simulink model "Flash_FCC"  (R2019b)
settings: Solver=FixedStepAuto  StartTime=0.0  StopTime=inf  RelTol=1e-3
undefined symbols (not defined in the file): Autopilot, AUX, den_lpf_d, dev, DiscIntNeverNeededParam, HIL_Data, num_lpf_d, pwm_output1
libraries: simulink_extras x4, px4lib x3, etargetslib x2, px4Sensorslib x1
settings Model: ExtModeTrigDuration=10  Creator=The MathWorks, Inc.  LastModifiedBy=guy-m
settings SolverCC: PositivePriorityOrder=on  AutoInsertRateTranBlk=on
settings OptimizationCC: EnhancedBackFolding=on  PassReuseOutputArgsAs=Individual arguments  MaxStackSize=64  OptimizeBlockOrder=speed  DifferentSizesBufferReuse=on  OptimizationCustomize=off  EfficientTunableParamExpr=on
settings DebuggingCC: InheritedTsInSrcMsg=none  ParameterTunabilityLossMsg=error
settings HardwareCC: ProdBitPerPointer=32  ProdBitPerSizeT=32  ProdBitPerPtrDiffT=32  ProdLargestAtomicInteger=Long  ProdLargestAtomicFloat=Double  ProdWordSize=32  ProdLongLongMode=on  ProdHWDeviceType=ARM Compatible->ARM Cortex
settings SFSimCC: MATLABDynamicMemAlloc=off  CustomCodeUndefinedFunction=UseInterfaceOnly
settings RTWCC: SystemTargetFile=ert.tlc  HardwareBoard=PX4 Pixhawk Series  TLCOptions="-aInlineSetEventsForThisBaseRateFcn=TLC_FALSE -aSuppressMultiTaskScheduler=TLC_FALSE  -aRateBasedStepFcn=0"  TemplateMakefile=ert_default_tmf  Toolchain=GNU Tools for PX4 Autopilots  IncludeHyperlinkInReport=on  TargetLang=C++
settings CodeAppCC: ForceParamTrailComments=on  IgnoreCustomStorageClasses=off  OperatorAnnotations=on  SimulinkDataObjDesc=on  SFDataObjDesc=on  InsertBlockDesc=on
settings ERTTargetCC: SupportContinuousTime=on  SupportVariableSizeSignals=on

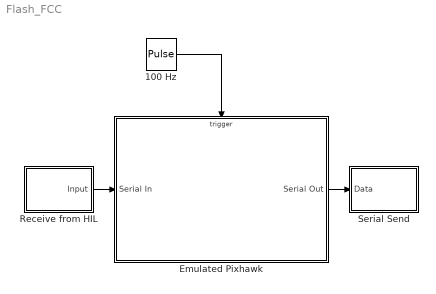
== system Flash_FCC ==
  100 Hz : DiscretePulseGenerator  PulseType=Time based  Period=0.01  PulseWidth=50
  Emulated Pixhawk : Subsystem
  Receive from HIL : Subsystem
  Serial Send : Subsystem
  wires:
  100 Hz/1 -> Emulated Pixhawk/Trigger
  Receive from HIL/1(Input) -> Emulated Pixhawk/1(Serial In)
  Emulated Pixhawk/1(Serial Out) -> Serial Send/1(Data)

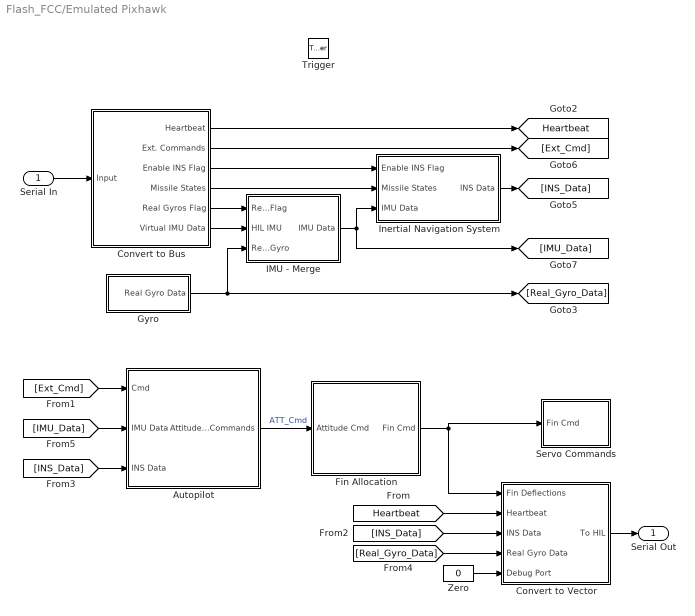
== system Flash_FCC/Emulated Pixhawk ==
  Serial In : Inport
  Trigger : TriggerPort  VariantControl=Variant  PortDimensions=1
  Autopilot : Subsystem
  Convert to Bus : Subsystem
  Convert to Vector : Subsystem
  Fin Allocation : Subsystem
  Gyro : Subsystem
  IMU - Merge : Subsystem
  Inertial Navigation System : Subsystem
  Servo Commands : Subsystem
  Zero : Constant  Value=0  OutDataTypeStr=Inherit: Inherit via back propagation
  Serial Out : Outport
  tag scope: Heartbeat=global
  wires:
  [Real_Gyro_Data] -> Convert to Vector/4(Real Gyro Data)
  Convert to Bus/2(Ext. Commands) -> [Ext_Cmd]
  Autopilot/1(Attitude_Commands) -> Fin Allocation/1(Attitude Cmd)  "ATT_Cmd"
  Convert to Bus/3(Enable INS Flag) -> Inertial Navigation System/1(Enable INS Flag)
  Inertial Navigation System/1(INS Data) -> [INS_Data]
  Zero/1 -> Convert to Vector/5(Debug Port)
  [Ext_Cmd] -> Autopilot/1(Cmd)
  [Heartbeat] -> Convert to Vector/2(Heartbeat)
  [IMU_Data] -> Autopilot/2(IMU Data)
  [INS_Data] -> Autopilot/3(INS Data)
  Gyro/1(Real Gyro Data) -> [Real_Gyro_Data], IMU - Merge/3(Real Gyro)
  IMU - Merge/1(IMU Data) -> [IMU_Data], Inertial Navigation System/3(IMU Data)
  Convert to Vector/1(To HIL) -> Serial Out/1
  Fin Allocation/1(Fin Cmd) -> Servo Commands/1(Fin Cmd), Convert to Vector/1(Fin Deflections)
  Serial In/1 -> Convert to Bus/1(Input)
  [INS_Data] -> Convert to Vector/3(INS Data)
  Convert to Bus/5(Real Gyros Flag) -> IMU - Merge/1(Real Gyro Flag)
  Convert to Bus/4(Missile States) -> Inertial Navigation System/2(Missile States)
  Convert to Bus/1(Heartbeat) -> [Heartbeat]
  Convert to Bus/6(Virtual IMU Data) -> IMU - Merge/2(HIL IMU)

== system Flash_FCC/Receive from HIL ==
  NOT : Logic  Operator=NOT  IconShape=distinctive  AllPortsSameDT=off  OutDataTypeStr=boolean
  Serial Receive : px4lib/Serial Receive  SCIModule=/dev/ttyACM0  DataType=single  DataLength=23  OutputStatus=on  SampleTime=0.001  BlockingMode=off  PartialData=off  Timeout=5
      settings: SourceProductName=Embedded Coder Support Package for PX4 Autopilots  SourceProductBaseCode=PX4AUTOPILOTS
  Triggered Subsystem : Subsystem  TreatAsAtomicUnit=on
  Input : Outport
  wires:
  Serial Receive/2 -> NOT/1
  NOT/1 -> Triggered Subsystem/Trigger
  Serial Receive/1 -> Triggered Subsystem/1(In1)
  Triggered Subsystem/1(Out1) -> Input/1

== system Flash_FCC/Serial Send ==
  Data : Inport
  Byte Pack : etargetslib/Byte Pack  datatypes={'single'}  byteAlign=1
      settings: SourceProductName=MATLAB Coder
  Header : Subsystem
  Serial Transmit : px4lib/Serial Transmit  SCIModule=/dev/ttyACM0
      settings: SourceProductName=Embedded Coder Support Package for PX4 Autopilots  SourceProductBaseCode=PX4AUTOPILOTS
  Vector Concatenate1 : Concatenate
  wires:
  Header/1(Out1) -> Vector Concatenate1/1
  Vector Concatenate1/1 -> Serial Transmit/1
  Byte Pack/1 -> Vector Concatenate1/2
  Data/1 -> Byte Pack/1

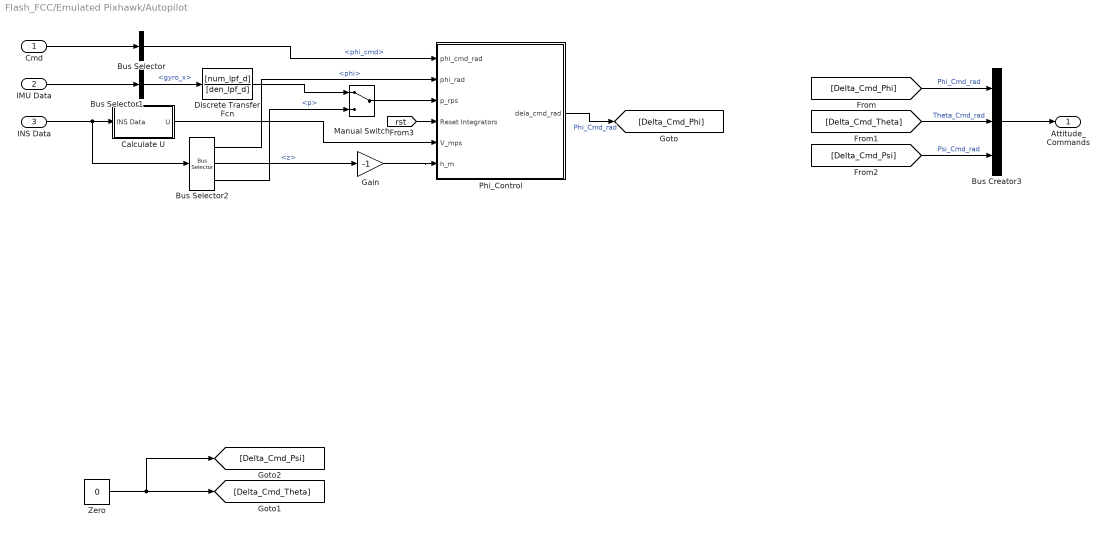
== system Flash_FCC/Emulated Pixhawk/Autopilot ==
  Cmd : Inport
  IMU Data : Inport  Port=2
  INS Data : Inport  Port=3
  Bus Creator3 : BusCreator  Inputs=3
  Bus Selector : BusSelector  OutputSignals=phi_cmd
  Bus Selector1 : BusSelector  OutputSignals=gyro_x
  Bus Selector2 : BusSelector  OutputSignals=phi,z,p
  Calculate U : Subsystem
  Discrete Transfer Fcn : DiscreteTransferFcn  Numerator=[num_lpf_d]  Denominator=[den_lpf_d]
  Gain : Gain  Gain=-1
  Manual Switch : ManualSwitch
  Phi_Control : Subsystem
  Zero : Constant  Value=0  OutDataTypeStr=Inherit: Inherit via back propagation
  Attitude_Commands : Outport  VectorParamsAs1DForOutWhenUnconnected=off
  wires:
  Bus Selector1/1 -> Discrete Transfer Fcn/1  "<gyro_x>"
  IMU Data/1 -> Bus Selector1/1
  Calculate U/1(U) -> Phi_Control/5(V_mps)
  Zero/1 -> [Delta_Cmd_Psi], [Delta_Cmd_Theta]
  [Delta_Cmd_Phi] -> Bus Creator3/1  "Phi_Cmd_rad"
  [Delta_Cmd_Theta] -> Bus Creator3/2  "Theta_Cmd_rad"
  Bus Creator3/1 -> Attitude_Commands/1
  [Delta_Cmd_Psi] -> Bus Creator3/3  "Psi_Cmd_rad"
  Bus Selector/1 -> Phi_Control/1(phi_cmd_rad)  "<phi_cmd>"
  Cmd/1 -> Bus Selector/1
  INS Data/1 -> Calculate U/1(INS Data), Bus Selector2/1
  Bus Selector2/1 -> Phi_Control/2(phi_rad)  "<phi>"
  [rst] -> Phi_Control/4(Reset Integrators)
  Bus Selector2/2 -> Gain/1  "<z>"
  Gain/1 -> Phi_Control/6(h_m)
  Phi_Control/1(dela_cmd_rad) -> [Delta_Cmd_Phi]  "Phi_Cmd_rad"
  Discrete Transfer Fcn/1 -> Manual Switch/1
  Bus Selector2/3 -> Manual Switch/2  "<p>"
  Manual Switch/1 -> Phi_Control/3(p_rps)

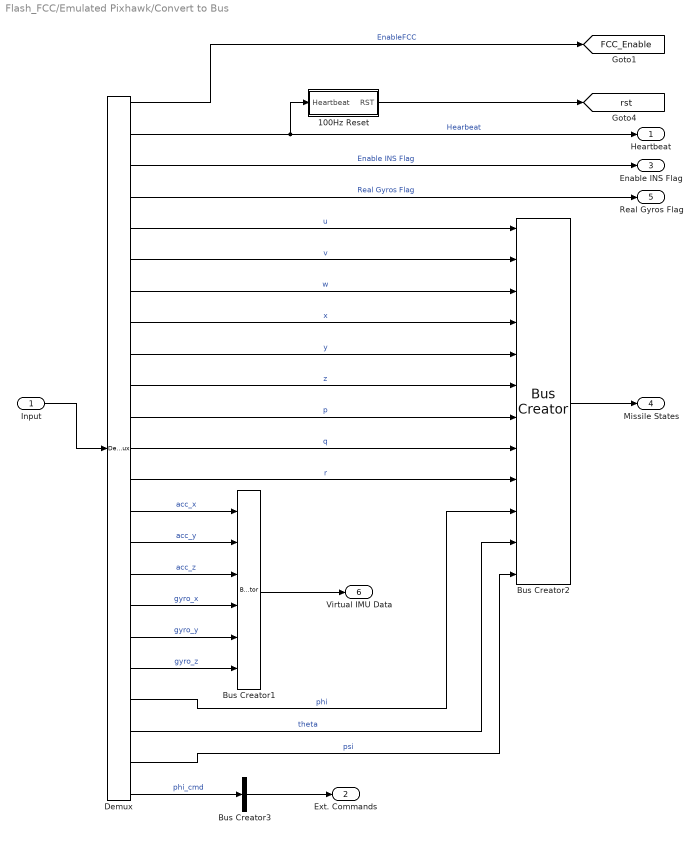
== system Flash_FCC/Emulated Pixhawk/Convert to Bus ==
  Input : Inport  OutDataTypeStr=single
  100Hz Reset : Subsystem
  Bus Creator1 : BusCreator  Inputs=6
  Bus Creator2 : BusCreator  Inputs=12
  Bus Creator3 : BusCreator  Inputs=1
  Demux : Demux  Outputs=23
  Heartbeat : Outport  InitialOutput=0
  Ext. Commands : Outport  Port=2  OutDataTypeStr=single  InitialOutput=0
  Enable INS Flag : Outport  Port=3  InitialOutput=0
  Missile States : Outport  Port=4  OutDataTypeStr=single  InitialOutput=[0 0 0 0 0 0 0 0 0 0]
  Real Gyros Flag : Outport  Port=5  InitialOutput=0
  Virtual IMU Data : Outport  Port=6  OutDataTypeStr=single  InitialOutput=[0 0 0 0 0 0 0 0 0 0]
  tag scope: FCC_Enable=global, rst=global
  wires:
  Demux/22 -> Bus Creator2/12  "psi"
  Demux/21 -> Bus Creator2/11  "theta"
  Demux/20 -> Bus Creator2/10  "phi"
  Demux/4 -> Real Gyros Flag/1  "Real Gyros Flag"
  Demux/5 -> Bus Creator2/1  "u"
  Demux/18 -> Bus Creator1/5  "gyro_y"
  Bus Creator1/1 -> Virtual IMU Data/1
  Demux/16 -> Bus Creator1/3  "acc_z"
  Demux/9 -> Bus Creator2/5  "y"
  Demux/14 -> Bus Creator1/1  "acc_x"
  Demux/17 -> Bus Creator1/4  "gyro_x"
  Demux/15 -> Bus Creator1/2  "acc_y"
  Demux/19 -> Bus Creator1/6  "gyro_z"
  Demux/12 -> Bus Creator2/8  "q"
  Demux/7 -> Bus Creator2/3  "w"
  Demux/10 -> Bus Creator2/6  "z"
  Demux/6 -> Bus Creator2/2  "v"
  Demux/11 -> Bus Creator2/7  "p"
  Demux/13 -> Bus Creator2/9  "r"
  Demux/23 -> Bus Creator3/1  "phi_cmd"
  Demux/8 -> Bus Creator2/4  "x"
  Bus Creator3/1 -> Ext. Commands/1
  Bus Creator2/1 -> Missile States/1
  Demux/1 -> [FCC_Enable]  "EnableFCC"
  Input/1 -> Demux/1
  Demux/2 -> 100Hz Reset/1(Heartbeat), Heartbeat/1  "Hearbeat"
  Demux/3 -> Enable INS Flag/1  "Enable INS Flag"
  100Hz Reset/1(RST) -> [rst]

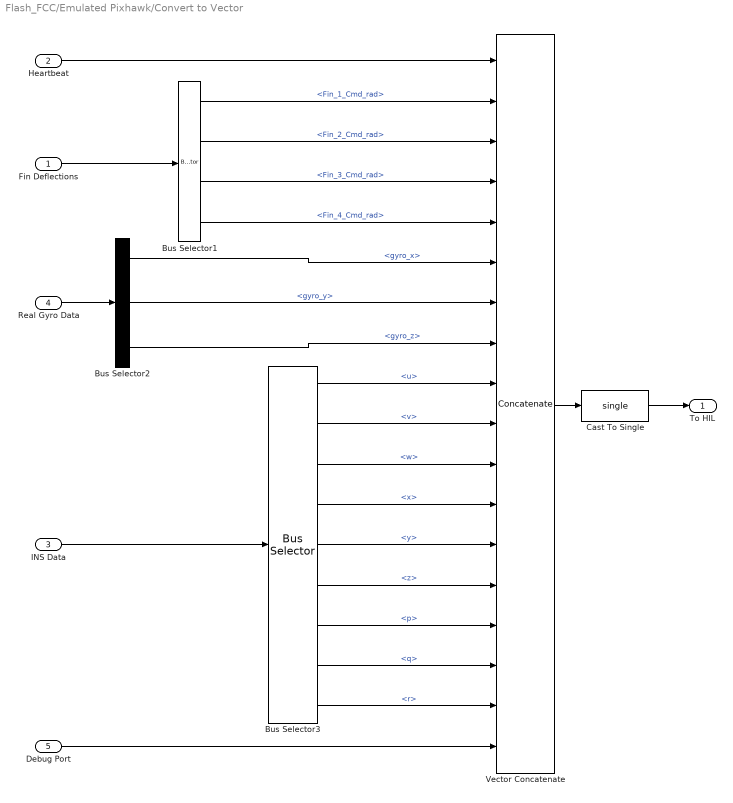
== system Flash_FCC/Emulated Pixhawk/Convert to Vector ==
  Fin Deflections : Inport
  Heartbeat : Inport  Port=2
  INS Data : Inport  Port=3
  Real Gyro Data : Inport  Port=4
  Debug Port : Inport  Port=5
  Bus Selector1 : BusSelector  OutputSignals=Fin_1_Cmd_rad,Fin_2_Cmd_rad,Fin_3_Cmd_rad,Fin_4_Cmd_rad
  Bus Selector2 : BusSelector  OutputSignals=gyro_x,gyro_y,gyro_z
  Bus Selector3 : BusSelector  OutputSignals=u,v,w,x,y,z,p,q,r
  Cast To Single : DataTypeConversion  OutDataTypeStr=single
  Vector Concatenate : Concatenate  NumInputs=18
  To HIL : Outport
  wires:
  Bus Selector1/3 -> Vector Concatenate/4  "<Fin_3_Cmd_rad>"
  Bus Selector1/4 -> Vector Concatenate/5  "<Fin_4_Cmd_rad>"
  Heartbeat/1 -> Vector Concatenate/1
  Bus Selector1/1 -> Vector Concatenate/2  "<Fin_1_Cmd_rad>"
  Bus Selector1/2 -> Vector Concatenate/3  "<Fin_2_Cmd_rad>"
  Vector Concatenate/1 -> Cast To Single/1
  Fin Deflections/1 -> Bus Selector1/1
  Cast To Single/1 -> To HIL/1
  Real Gyro Data/1 -> Bus Selector2/1
  Bus Selector3/7 -> Vector Concatenate/15  "<p>"
  Bus Selector3/5 -> Vector Concatenate/13  "<y>"
  Bus Selector3/4 -> Vector Concatenate/12  "<x>"
  Bus Selector3/9 -> Vector Concatenate/17  "<r>"
  Bus Selector3/3 -> Vector Concatenate/11  "<w>"
  Bus Selector2/3 -> Vector Concatenate/8  "<gyro_z>"
  Debug Port/1 -> Vector Concatenate/18
  Bus Selector3/1 -> Vector Concatenate/9  "<u>"
  Bus Selector2/2 -> Vector Concatenate/7  "<gyro_y>"
  Bus Selector2/1 -> Vector Concatenate/6  "<gyro_x>"
  Bus Selector3/8 -> Vector Concatenate/16  "<q>"
  INS Data/1 -> Bus Selector3/1
  Bus Selector3/6 -> Vector Concatenate/14  "<z>"
  Bus Selector3/2 -> Vector Concatenate/10  "<v>"

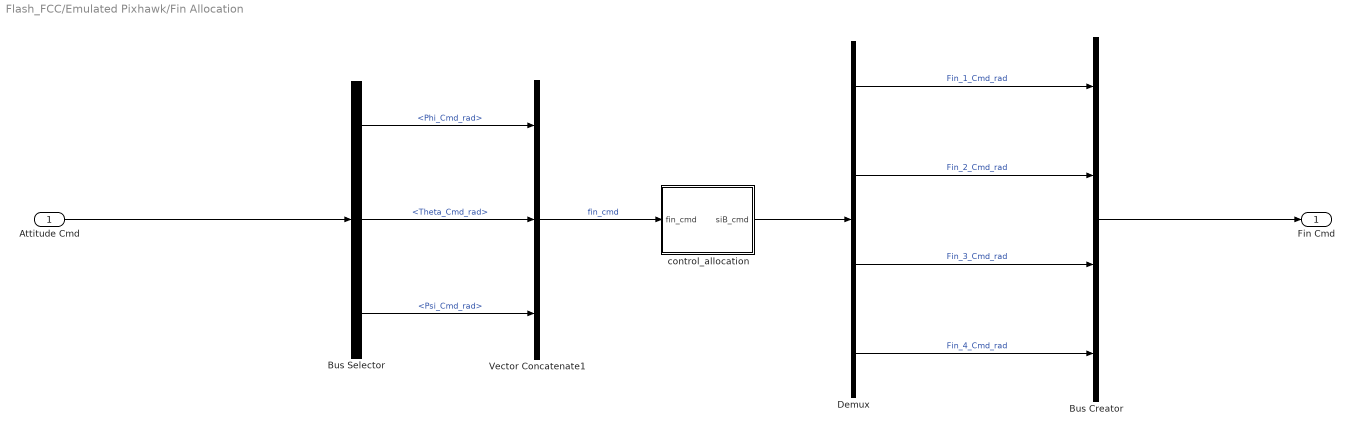
== system Flash_FCC/Emulated Pixhawk/Fin Allocation ==
  Attitude Cmd : Inport
  Bus Creator : BusCreator  Inputs=4
  Bus Selector : BusSelector  OutputSignals=Phi_Cmd_rad,Theta_Cmd_rad,Psi_Cmd_rad
  Demux : Demux
  Vector Concatenate1 : Concatenate  NumInputs=3
  control_allocation : Subsystem
  Fin Cmd : Outport  VectorParamsAs1DForOutWhenUnconnected=off
  wires:
  Demux/4 -> Bus Creator/4  "Fin_4_Cmd_rad"
  control_allocation/1(siB_cmd) -> Demux/1
  Bus Selector/3 -> Vector Concatenate1/3  "<Psi_Cmd_rad>"
  Vector Concatenate1/1 -> control_allocation/1(fin_cmd)  "fin_cmd"
  Bus Selector/1 -> Vector Concatenate1/1  "<Phi_Cmd_rad>"
  Demux/3 -> Bus Creator/3  "Fin_3_Cmd_rad"
  Bus Selector/2 -> Vector Concatenate1/2  "<Theta_Cmd_rad>"
  Demux/1 -> Bus Creator/1  "Fin_1_Cmd_rad"
  Bus Creator/1 -> Fin Cmd/1
  Attitude Cmd/1 -> Bus Selector/1
  Demux/2 -> Bus Creator/2  "Fin_2_Cmd_rad"

== system Flash_FCC/Emulated Pixhawk/Gyro ==
  Bus Creator2 : BusCreator  Inputs=3
  Gyroscope : px4Sensorslib/Gyroscope  uorbTimeStamp=off  BlockingMode=off  BlockTimeout=1e-3  sampleTime=-1
      settings: SourceProductName=Embedded Coder Support Package for PX4 Autopilots  SourceProductBaseCode=PX4AUTOPILOTS
  Terminator3 : Terminator
  Real Gyro Data : Outport
  wires:
  Gyroscope/1 -> Terminator3/1
  Bus Creator2/1 -> Real Gyro Data/1  "gyro"
  Gyroscope/4 -> Bus Creator2/3  "gyro_z"
  Gyroscope/2 -> Bus Creator2/1  "gyro_x"
  Gyroscope/3 -> Bus Creator2/2  "gyro_y"

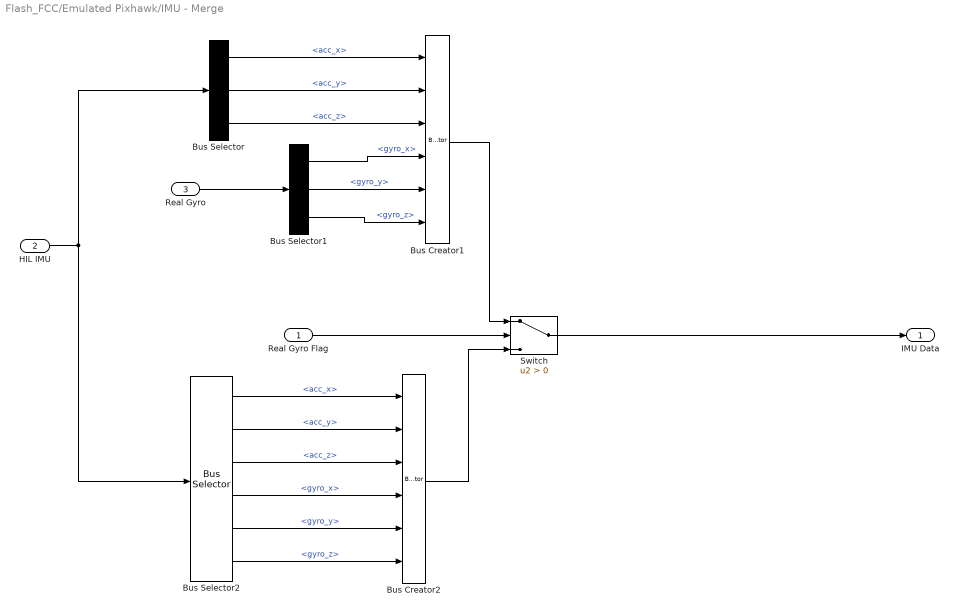
== system Flash_FCC/Emulated Pixhawk/IMU - Merge ==
  Real Gyro Flag : Inport
  HIL IMU : Inport  Port=2
  Real Gyro : Inport  Port=3
  Bus Creator1 : BusCreator  Inputs=6
  Bus Creator2 : BusCreator  Inputs=6
  Bus Selector : BusSelector  OutputSignals=acc_x,acc_y,acc_z
  Bus Selector1 : BusSelector  OutputSignals=gyro_x,gyro_y,gyro_z
  Bus Selector2 : BusSelector  OutputSignals=acc_x,acc_y,acc_z,gyro_x,gyro_y,gyro_z
  Switch : Switch  Criteria=u2 > Threshold
  IMU Data : Outport
  wires:
  Real Gyro Flag/1 -> Switch/2
  Real Gyro/1 -> Bus Selector1/1
  HIL IMU/1 -> Bus Selector2/1, Bus Selector/1
  Bus Selector/3 -> Bus Creator1/3  "<acc_z>"
  Bus Selector/1 -> Bus Creator1/1  "<acc_x>"
  Bus Selector/2 -> Bus Creator1/2  "<acc_y>"
  Bus Selector1/1 -> Bus Creator1/4  "<gyro_x>"
  Bus Selector1/3 -> Bus Creator1/6  "<gyro_z>"
  Bus Creator1/1 -> Switch/1
  Bus Selector1/2 -> Bus Creator1/5  "<gyro_y>"
  Bus Selector2/5 -> Bus Creator2/5  "<gyro_y>"
  Bus Selector2/6 -> Bus Creator2/6  "<gyro_z>"
  Bus Selector2/4 -> Bus Creator2/4  "<gyro_x>"
  Bus Selector2/2 -> Bus Creator2/2  "<acc_y>"
  Bus Selector2/1 -> Bus Creator2/1  "<acc_x>"
  Bus Selector2/3 -> Bus Creator2/3  "<acc_z>"
  Bus Creator2/1 -> Switch/3
  Switch/1 -> IMU Data/1

== system Flash_FCC/Emulated Pixhawk/Inertial Navigation System ==
  Enable INS Flag : Inport
  Missile States : Inport  Port=2
  IMU Data : Inport  Port=3
  INS (INCOMPLETE) : Subsystem
  Switch : Switch  Criteria=u2 > Threshold
  INS Data : Outport
  wires:
  Enable INS Flag/1 -> Switch/2
  IMU Data/1 -> INS (INCOMPLETE)/1(IMU Data)
  Switch/1 -> INS Data/1
  Missile States/1 -> Switch/3
  INS (INCOMPLETE)/1(INS Data) -> Switch/1

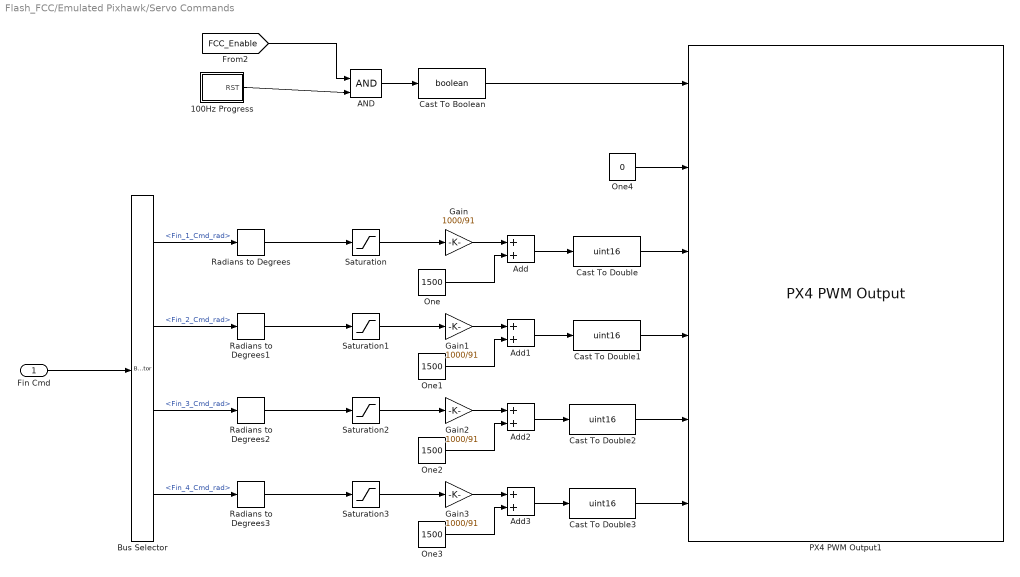
== system Flash_FCC/Emulated Pixhawk/Servo Commands ==
  Fin Cmd : Inport
  100Hz Progress : Subsystem
  AND : Logic  IconShape=distinctive  AllPortsSameDT=off  OutDataTypeStr=boolean
  Add{,1..3} (4 alike) : Sum
  Bus Selector : BusSelector  OutputSignals=Fin_1_Cmd_rad,Fin_2_Cmd_rad,Fin_3_Cmd_rad,Fin_4_Cmd_rad
  Cast To Boolean : DataTypeConversion  OutDataTypeStr=boolean
  Cast To Double{,1..3} (4 alike) : DataTypeConversion  OutDataTypeStr=uint16
  Gain{,1..3} (4 alike) : Gain  Gain=1000/91
  One{,1..3} (4 alike) : Constant  Value=1500  OutDataTypeStr=Inherit: Inherit via back propagation
  One4 : Constant  Value=0  OutDataTypeStr=boolean
  PX4 PWM Output1 : px4lib/PX4 PWM Output  pwmDevice=AUX (/dev/pwm_output1)  pwmChannel1_=on  pwmChannel2_=on  pwmChannel3_=on  pwmChannel4_=on  pwmChannel5_=off  pwmChannel6_=off  pwmChannel7_=off  pwmChannel8_=off  forceTerminateFailsafe=off  outputErrorStatus=off
      settings: SourceProductName=Embedded Coder Support Package for PX4 Autopilots  SourceProductBaseCode=PX4AUTOPILOTS
  Radians to Degrees{,1..3} (4 alike) : simulink_extras/Transformations/Radians to Degrees
  Saturation{,1..3} (4 alike) : Saturate  UpperLimit=20  LowerLimit=-20
  wires:
  Saturation2/1 -> Gain2/1
  Cast To Double3/1 -> PX4 PWM Output1/6
  One4/1 -> PX4 PWM Output1/2
  One/1 -> Add/2
  One2/1 -> Add2/2
  Add1/1 -> Cast To Double1/1
  Gain2/1 -> Add2/1
  AND/1 -> Cast To Boolean/1
  Radians to Degrees1/1 -> Saturation1/1
  Cast To Double2/1 -> PX4 PWM Output1/5
  Add2/1 -> Cast To Double2/1
  Fin Cmd/1 -> Bus Selector/1
  Cast To Double1/1 -> PX4 PWM Output1/4
  Bus Selector/2 -> Radians to Degrees1/1  "<Fin_2_Cmd_rad>"
  Gain/1 -> Add/1
  Bus Selector/4 -> Radians to Degrees3/1  "<Fin_4_Cmd_rad>"
  One3/1 -> Add3/2
  Saturation/1 -> Gain/1
  Gain1/1 -> Add1/1
  Saturation3/1 -> Gain3/1
  Gain3/1 -> Add3/1
  Radians to Degrees3/1 -> Saturation3/1
  Bus Selector/1 -> Radians to Degrees/1  "<Fin_1_Cmd_rad>"
  Bus Selector/3 -> Radians to Degrees2/1  "<Fin_3_Cmd_rad>"
  Saturation1/1 -> Gain1/1
  Cast To Double/1 -> PX4 PWM Output1/3
  Add3/1 -> Cast To Double3/1
  Radians to Degrees2/1 -> Saturation2/1
  [FCC_Enable] -> AND/1
  Radians to Degrees/1 -> Saturation/1
  100Hz Progress/1(RST) -> AND/2
  One1/1 -> Add1/2
  Add/1 -> Cast To Double/1
  Cast To Boolean/1 -> PX4 PWM Output1/1

== system Flash_FCC/Receive from HIL/Triggered Subsystem ==
  In1 : Inport
  Trigger : TriggerPort  VariantControl=Variant
  Out1 : Outport  InitialOutput=0
  wires:
  In1/1 -> Out1/1

== system Flash_FCC/Serial Send/Header ==
  note: Serial header - used to preserve order of bytes
  Byte Pack1 : etargetslib/Byte Pack  datatypes={'uint8'}  byteAlign=1
      settings: SourceProductName=MATLAB Coder
  Zero : Constant  Value=[5 5 5]  OutDataTypeStr=uint8  SampleTime=-1
  Out1 : Outport
  wires:
  Zero/1 -> Byte Pack1/1
  Byte Pack1/1 -> Out1/1

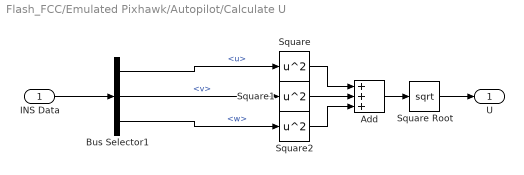
== system Flash_FCC/Emulated Pixhawk/Autopilot/Calculate U ==
  INS Data : Inport
  Add : Sum  Inputs=+++
  Bus Selector1 : BusSelector  OutputSignals=u,v,w
  Square : Math  Operator=square  SignedPower=off  SaturateOnIntegerOverflow=on
  Square Root : Sqrt  SaturateOnIntegerOverflow=on
  Square1 : Math  Operator=square  SignedPower=off  SaturateOnIntegerOverflow=on
  Square2 : Math  Operator=square  SignedPower=off  SaturateOnIntegerOverflow=on
  U : Outport
  wires:
  Square/1 -> Add/1
  Square2/1 -> Add/3
  Square Root/1 -> U/1
  Add/1 -> Square Root/1
  Square1/1 -> Add/2
  Bus Selector1/2 -> Square1/1  "<v>"
  Bus Selector1/3 -> Square2/1  "<w>"
  Bus Selector1/1 -> Square/1  "<u>"
  INS Data/1 -> Bus Selector1/1

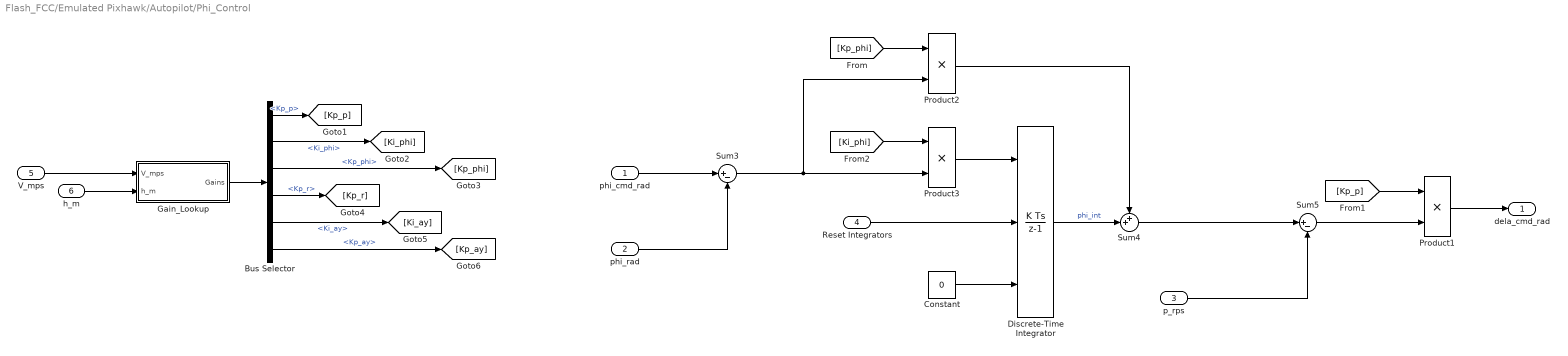
== system Flash_FCC/Emulated Pixhawk/Autopilot/Phi_Control ==
  phi_cmd_rad : Inport
  phi_rad : Inport  Port=2
  p_rps : Inport  Port=3
  Reset Integrators : Inport  Port=4
  V_mps : Inport  Port=5
  h_m : Inport  Port=6
  Bus Selector : BusSelector  OutputSignals=Kp_p,Ki_phi,Kp_phi,Kp_r,Ki_ay,Kp_ay
  Constant : Constant  Value=0  OutDataTypeStr=single
  Discrete-Time Integrator : DiscreteIntegrator  ExternalReset=level  InitialConditionSource=external  SampleTime=-1  OutDataTypeStr=single  ICPrevOutput=DiscIntNeverNeededParam  ICPrevScaledInput=DiscIntNeverNeededParam
  Gain_Lookup : Subsystem
  Product1 : Product
  Product2 : Product
  Product3 : Product
  Sum3 : Sum  Inputs=|+-
  Sum4 : Sum  Inputs=++|
  Sum5 : Sum  Inputs=|+-
  dela_cmd_rad : Outport
  wires:
  phi_cmd_rad/1 -> Sum3/1
  Reset Integrators/1 -> Discrete-Time Integrator/2
  p_rps/1 -> Sum5/2
  phi_rad/1 -> Sum3/2
  Product2/1 -> Sum4/1
  Sum3/1 -> Product3/2, Product2/2
  Constant/1 -> Discrete-Time Integrator/3
  Sum5/1 -> Product1/2
  [Ki_phi] -> Product3/1
  Product1/1 -> dela_cmd_rad/1
  [Kp_p] -> Product1/1
  [Kp_phi] -> Product2/1
  Discrete-Time Integrator/1 -> Sum4/2  "phi_int"
  Sum4/1 -> Sum5/1
  Product3/1 -> Discrete-Time Integrator/1
  h_m/1 -> Gain_Lookup/2(h_m)
  Bus Selector/6 -> [Kp_ay]  "<Kp_ay>"
  Bus Selector/5 -> [Ki_ay]  "<Ki_ay>"
  Bus Selector/2 -> [Ki_phi]  "<Ki_phi>"
  Bus Selector/1 -> [Kp_p]  "<Kp_p>"
  V_mps/1 -> Gain_Lookup/1(V_mps)
  Bus Selector/4 -> [Kp_r]  "<Kp_r>"
  Gain_Lookup/1(Gains) -> Bus Selector/1
  Bus Selector/3 -> [Kp_phi]  "<Kp_phi>"

== system Flash_FCC/Emulated Pixhawk/Convert to Bus/100Hz Reset ==
  Heartbeat : Inport
  Delay : Delay  DelayLength=1
  GreaterThan : RelationalOperator  Operator=<  OutDataTypeStr=boolean  RndMeth=Simplest
  RST : Outport
  wires:
  GreaterThan/1 -> RST/1
  Delay/1 -> GreaterThan/2
  Heartbeat/1 -> Delay/1, GreaterThan/1

== system Flash_FCC/Emulated Pixhawk/Fin Allocation/control_allocation ==
  fin_cmd : Inport
  Constant7 : Constant  Value=HIL_Data.FDM.Tr4r3  OutDataTypeStr=single
  Product : Product  Multiplication=Matrix(*)
  siB_cmd : Outport  VectorParamsAs1DForOutWhenUnconnected=off
  wires:
  Constant7/1 -> Product/1
  fin_cmd/1 -> Product/2
  Product/1 -> siB_cmd/1  "siB_cmd"

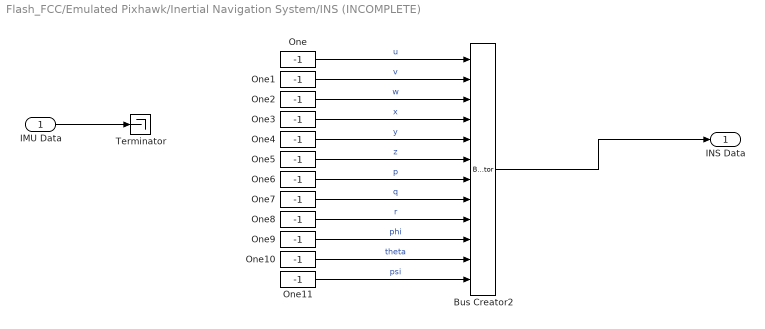
== system Flash_FCC/Emulated Pixhawk/Inertial Navigation System/INS (INCOMPLETE) ==
  IMU Data : Inport
  Bus Creator2 : BusCreator  Inputs=12
  One{,1..11} (12 alike) : Constant  Value=-1  OutDataTypeStr=Inherit: Inherit via back propagation
  Terminator : Terminator
  INS Data : Outport
  wires:
  One11/1 -> Bus Creator2/12  "psi"
  One10/1 -> Bus Creator2/11  "theta"
  One9/1 -> Bus Creator2/10  "phi"
  One8/1 -> Bus Creator2/9  "r"
  One7/1 -> Bus Creator2/8  "q"
  One2/1 -> Bus Creator2/3  "w"
  One6/1 -> Bus Creator2/7  "p"
  One4/1 -> Bus Creator2/5  "y"
  One1/1 -> Bus Creator2/2  "v"
  One5/1 -> Bus Creator2/6  "z"
  One/1 -> Bus Creator2/1  "u"
  One3/1 -> Bus Creator2/4  "x"
  IMU Data/1 -> Terminator/1
  Bus Creator2/1 -> INS Data/1

== system Flash_FCC/Emulated Pixhawk/Servo Commands/100Hz Progress ==
  Delay : Delay  DelayLength=1
  GreaterThan : RelationalOperator  Operator=>  OutDataTypeStr=boolean  RndMeth=Simplest
  RST : Outport
  wires:
  GreaterThan/1 -> RST/1
  Delay/1 -> GreaterThan/2
  [Heartbeat] -> Delay/1, GreaterThan/1

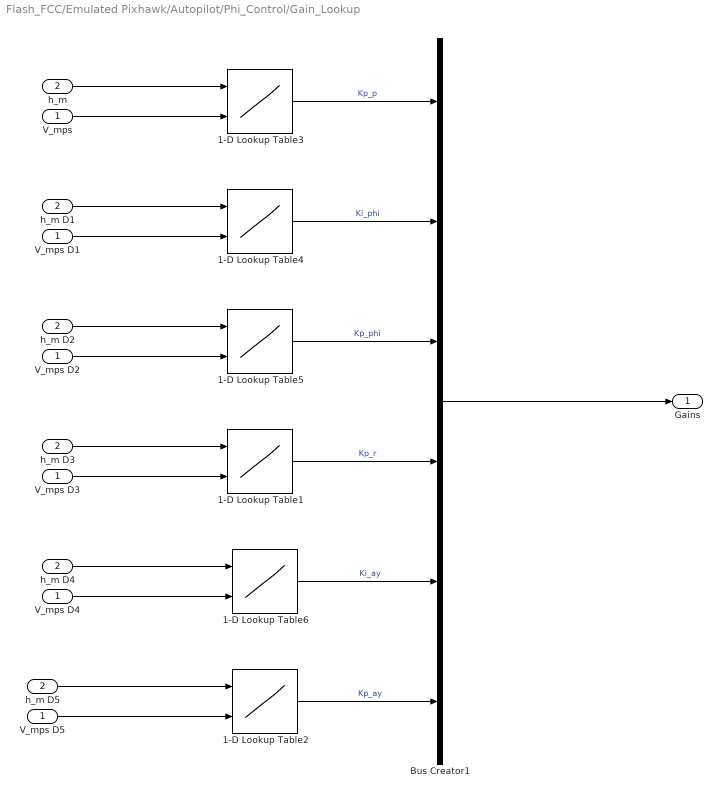
== system Flash_FCC/Emulated Pixhawk/Autopilot/Phi_Control/Gain_Lookup ==
  V_mps : Inport
  h_m : Inport  Port=2
  1-D Lookup Table1 : Lookup_n-D  BreakpointsForDimension1=Autopilot.Ay.h_bkpts_m  BreakpointsForDimension2=Autopilot.Ay.V_bkpts_mps  Table=Autopilot.Ay.Kp_r_vec  ExtrapMethod=Clip  UseLastTableValue=on  InternalRulePriority=Speed  RndMeth=Simplest  InputSameDT=on
      settings: AttributesFormatString=|
      | %<Table>
      | %<BreakpointsForDimension1>
      | %<BreakpointsForDimension2>
  1-D Lookup Table2 : Lookup_n-D  BreakpointsForDimension1=Autopilot.Ay.h_bkpts_m  BreakpointsForDimension2=Autopilot.Ay.V_bkpts_mps  Table=Autopilot.Ay.Kp_ay_vec  ExtrapMethod=Clip  UseLastTableValue=on  InternalRulePriority=Speed  RndMeth=Simplest  InputSameDT=on
      settings: AttributesFormatString=|
      | %<Table>
      | %<BreakpointsForDimension1>
      | %<BreakpointsForDimension2>
  1-D Lookup Table3 : Lookup_n-D  BreakpointsForDimension1=Autopilot.Phi.h_bkpts_m  BreakpointsForDimension2=Autopilot.Phi.V_bkpts_mps  Table=Autopilot.Phi.Kp_p_vec  ExtrapMethod=Clip  UseLastTableValue=on  InternalRulePriority=Speed  RndMeth=Simplest  InputSameDT=on
      settings: AttributesFormatString=|
      | %<Table>
      | %<BreakpointsForDimension1>
      | %<BreakpointsForDimension2>
  1-D Lookup Table4 : Lookup_n-D  BreakpointsForDimension1=Autopilot.Phi.h_bkpts_m  BreakpointsForDimension2=Autopilot.Phi.V_bkpts_mps  Table=Autopilot.Phi.Ki_phi_vec  ExtrapMethod=Clip  UseLastTableValue=on  InternalRulePriority=Speed  RndMeth=Simplest  InputSameDT=on
      settings: AttributesFormatString=|
      | %<Table>
      | %<BreakpointsForDimension1>
      | %<BreakpointsForDimension2>
  1-D Lookup Table5 : Lookup_n-D  BreakpointsForDimension1=Autopilot.Phi.h_bkpts_m  BreakpointsForDimension2=Autopilot.Phi.V_bkpts_mps  Table=Autopilot.Phi.Kp_phi_vec  ExtrapMethod=Clip  UseLastTableValue=on  InternalRulePriority=Speed  RndMeth=Simplest  InputSameDT=on
      settings: AttributesFormatString=|
      | %<Table>
      | %<BreakpointsForDimension1>
      | %<BreakpointsForDimension2>
  1-D Lookup Table6 : Lookup_n-D  BreakpointsForDimension1=Autopilot.Ay.h_bkpts_m  BreakpointsForDimension2=Autopilot.Ay.V_bkpts_mps  Table=Autopilot.Ay.Ki_ay_vec  ExtrapMethod=Clip  UseLastTableValue=on  InternalRulePriority=Speed  RndMeth=Simplest  InputSameDT=on
      settings: AttributesFormatString=|
      | %<Table>
      | %<BreakpointsForDimension1>
      | %<BreakpointsForDimension2>
  Bus Creator1 : BusCreator  Inputs=6
  V_mps D{1..5} (5 alike) : InportShadow
  h_m D{1..5} (5 alike) : InportShadow  Port=2
  Gains : Outport
  wires:
  h_m/1 -> 1-D Lookup Table3/1
  Bus Creator1/1 -> Gains/1
  1-D Lookup Table5/1 -> Bus Creator1/3  "Kp_phi"
  1-D Lookup Table4/1 -> Bus Creator1/2  "Ki_phi"
  1-D Lookup Table3/1 -> Bus Creator1/1  "Kp_p"
  V_mps/1 -> 1-D Lookup Table3/2
  h_m D1/1 -> 1-D Lookup Table4/1
  V_mps D1/1 -> 1-D Lookup Table4/2
  h_m D2/1 -> 1-D Lookup Table5/1
  V_mps D2/1 -> 1-D Lookup Table5/2
  1-D Lookup Table2/1 -> Bus Creator1/6  "Kp_ay"
  1-D Lookup Table6/1 -> Bus Creator1/5  "Ki_ay"
  1-D Lookup Table1/1 -> Bus Creator1/4  "Kp_r"
  h_m D3/1 -> 1-D Lookup Table1/1
  V_mps D3/1 -> 1-D Lookup Table1/2
  h_m D4/1 -> 1-D Lookup Table6/1
  V_mps D4/1 -> 1-D Lookup Table6/2
  h_m D5/1 -> 1-D Lookup Table2/1
  V_mps D5/1 -> 1-D Lookup Table2/2
